simulink model "satellite_sim"  (R2019b)
settings: Solver=ode45  StartTime=0.0  StopTime=10000  RelTol=1e-3  EnableMultiTasking=on
InitFcn:
  | restoredefaultpath
  | clear all
  | addpath('./..')
  | satellite_param
undefined symbols (not defined in the file or in its folder): P, satellite_animation
libraries: simulink x2
settings Model: Creator=beard  LastModifiedBy=JoHn
settings DataIOCC: LimitDataPoints=on  SaveFormat=Array  SignalLoggingSaveFormat=ModelDataLogs  ReturnWorkspaceOutputs=off
settings OptimizationCC: ExpressionDepthLimit=2147483647  InitFltsAndDblsToZero=on  LifeSpan=inf
settings DebuggingCC: UnderspecifiedInitializationDetection=Classic  MergeDetectMultiDrivingBlocksExec=none  SolverPrmCheckMsg=warning  FcnCallInpInsideContextMsg=warning  StateNameClashWarn=warning  SFUnexpectedBacktrackingDiag=warning  SFNoUnconditionalDefaultTransitionDiag=warning  SFExecutionAtInitializationDiag=none  ArithmeticOperatorsInVariantConditions=warning
settings HardwareCC: ProdBitPerPointer=32  ProdBitPerSizeT=32  ProdBitPerPtrDiffT=32  ProdLargestAtomicFloat=None  ProdIntDivRoundTo=Undefined  ProdEndianess=Unspecified  ProdWordSize=32  ProdHWDeviceType=32-bit Generic
settings ModelReferenceCC: PropagateSignalLabelsOutOfModel=off
settings SFSimCC: SimUseLocalCustomCode=off  CustomCodeUndefinedFunction=UseInterfaceOnly
settings RTWCC: RTWUseLocalCustomCode=off
settings CodeAppCC: StateflowObjectComments=on
settings GRTTargetCC: TargetLangStandard=C89/C90 (ANSI)  GeneratePreprocessorConditionals=Disable all  CombineOutputUpdateFcns=off  GRTInterface=on
settings ConfigComp: CovMetricSettings=dw  CovHtmlReporting=on  CovSaveCumulativeToWorkspaceVar=on  CovSaveSingleToWorkspaceVar=on  CovExternalEMLEnable=off

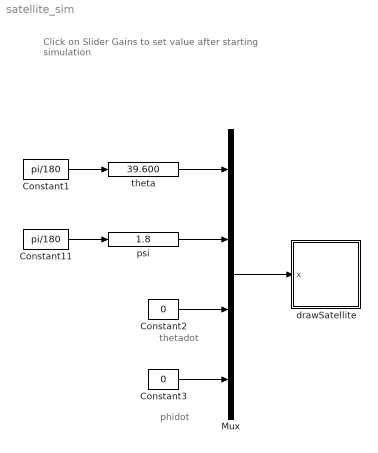
== system satellite_sim ==
  note: phidot
  note: thetadot
  note: Click on Slider Gains to set value
      | after starting simulation
  Constant1 : Constant  Value=pi/180
  Constant11 : Constant  Value=pi/180
  Constant2 : Constant  Value=0
  Constant3 : Constant  Value=0
  Mux : Mux
  drawSatellite : Subsystem
      mask Display: image(imread('tv.jpg'))
  psi : simulink/Math Operations/Slider Gain  gain=1.8  low=-90  high=90
  theta : simulink/Math Operations/Slider Gain  gain=39.600  low=-180  high=180
  wires:
  theta/1 -> Mux/1
  psi/1 -> Mux/2
  Constant11/1 -> psi/1
  Mux/1 -> drawSatellite/1(x)
  Constant1/1 -> theta/1
  Constant2/1 -> Mux/3
  Constant3/1 -> Mux/4

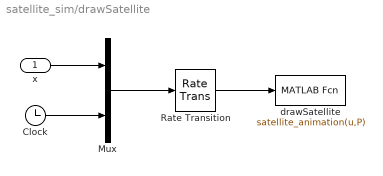
== system satellite_sim/drawSatellite ==
  x : Inport
  Clock : Clock
  Mux : Mux  Inputs=2
  Rate Transition : RateTransition  OutPortSampleTime=P.t_plot
  drawSatellite : MATLABFcn  MATLABFcn=satellite_animation(u,P)  OutputDimensions=0
  wires:
  Mux/1 -> Rate Transition/1
  x/1 -> Mux/1
  Clock/1 -> Mux/2
  Rate Transition/1 -> drawSatellite/1
